simulink model "bidirectional_fixvoltage"  (R2016a)
settings: Solver=ode1  StartTime=0.0  StopTime=inf  FixedStep=1e-5  RelTol=1e-3
undefined symbols (not defined in the file): Ion, Lithium
libraries: powerlib x12, simulink x2, electricdrivelib x1
settings Model: Creator=Power Lab  LastModifiedBy=VARUN SINGH
settings DataIOCC: LimitDataPoints=on
settings DebuggingCC: AllowSymbolicDim=off
settings ModelReferenceCC: PropagateSignalLabelsOutOfModel=off
settings GRTTargetCC: GeneratePreprocessorConditionals=Use local settings

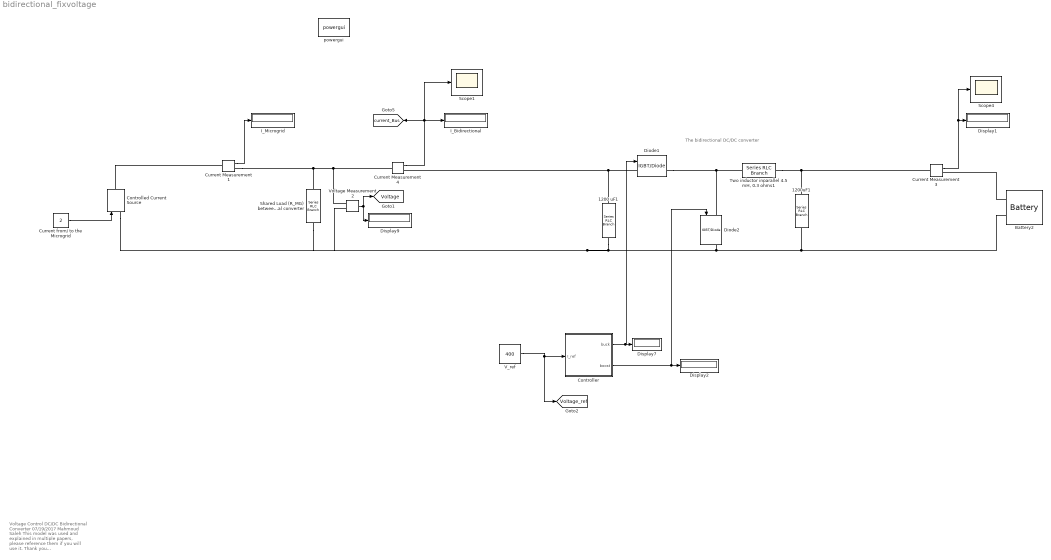
== system bidirectional_fixvoltage ==
  note: Voltage Control DC/DC Bidirectional Converter
      | 07/19/2017 Mahmoud Saleh
      | This model was used and explained in multiple papers, please reference them if you will use it. Thank you
      | ---------------------------------------------------------------------------------------------------------------------------------------------------
      |
      | http://ieeexplore.ieee.org/document/7454295/
      | OR: https://drive.google.com/open?id=0B7mblFaJhY4VcmZ5OF9ueGxPM1U
      |
      | For Citation use :
      | - M. Saleh , Y. Esa, Y. Mhandi, W. Brandauer and A. Mohamed, "Design and implementation of CCNY DC microgrid testbed,"
      | 2016 IEEE Industry Applications Society Annual Meeting, Portland, OR, 2016.
      |
      | Also This Model was used in the paper:
      | http://ieeexplore.ieee.org/abstract/document/7731870/
      | OR: https://drive.google.com/open?id=0B7mblFaJhY4VY0dXdWdqTWNmUDg
      |
      | For Citation use :
      | -M. Saleh , A. Althaibani, Y. Esa, Y. Mhandi and A. Mohamed, "Impact of clustering microgrids on their stability and resilience during blackouts,"
      | 2015 International Conference on Smart Grid and Clean Energy Technologies (ICSGCE), Offenburg, 2015, pp. 195-200.
      |
      | Also was used in the following paper:
      | https://drive.google.com/open?id=0B7mblFaJhY4VclFOR2dLcEhQYmc
      |
      | M. Saleh, Y. Esa, and A. Moahmed “Centralized Control for DC Microgrid Using Finite State Machine” accepted and to presented
      | at the 2017 IEEE Innovative Smart Grid Technologies Conference (ISGT), Washington D.C. Metro Area, USA, 23-26 April 2017.
  note: The bidirectional DC/DC converter
  1200 uF1 : powerlib/Elements/Series RLC Branch  LConnTagsString=__new0  RConnTagsString=__new0  BranchType=RC  Resistance=0.001  Inductance=3e-3  SetiL0=off  InitialCurrent=0  Capacitance=1200e-6  Setx0=off  InitialVoltage=0  Measurements=None
  1200uF1 : powerlib/Elements/Series RLC Branch  LConnTagsString=__new0  RConnTagsString=__new0  BranchType=C  Resistance=1  Inductance=3e-3  SetiL0=off  InitialCurrent=0  Capacitance=1200e-6  Setx0=off  InitialVoltage=0  Measurements=None
  Battery2 : electricdrivelib/Extra Sources/Battery  BatType=Lithium-Ion  ShowTempParam=off  ThermalPreset=no  NomV=120  NomQ=100  SOC=50  Batt_Tr=0.1  PresetModel=on  MaxQ=100  MinV=90  FullV=139.6785  Dis_rate=43.4783  R=0.012  Normal_OP=90.4348  expZone="[129.6463      4.913043]"  current=[1.5 3]  Units=Ampere-hour  Tci=20  NomT=20  T2=-30  MaxQ2=4.8  FullV2=7.1  Normal_OP2=5.72  expZone2="[6.58  1]"  Rca=0.6  ti=1000  Dp=0
  Controlled Current Source : powerlib/Electrical Sources/Controlled Current Source  Initialize=on  Source_Type=AC  Amplitude=0  Phase=0  Frequency=0  Measurements=None
  Controller : Subsystem
  Current Measurement1 : powerlib/Measurements/Current Measurement  PhasorSimulation=off  OutputType=Complex  PSBequivalent=0
  Current Measurement3 : powerlib/Measurements/Current Measurement  PhasorSimulation=off  OutputType=Complex  PSBequivalent=0
  Current Measurement4 : powerlib/Measurements/Current Measurement  PhasorSimulation=off  OutputType=Complex  PSBequivalent=0
  Current from/ to the Microgrid : Constant  Value=2
  Diode1 : powerlib/Power Electronics/IGBT//Diode  Ron=1e-3  Rs=1e5  Cs=inf  Measurements=on
  Diode2 : powerlib/Power Electronics/IGBT//Diode  Ron=1e-3  Rs=1e5  Cs=inf  Measurements=on
  Display{1..2,7,9} (4 alike) : Display
  I_Bidirectional : Display
  I_Microgrid : Display
  Scope1 : Scope
  Scope4 : Scope
  "Shared Load (R_MG) between the Microgrid and the battery through the bidirectional converter " : powerlib/Elements/Series RLC Branch  LConnTagsString=__new0  RConnTagsString=__new0  BranchType=R  Resistance=100  Inductance=3e-3  SetiL0=off  InitialCurrent=0  Capacitance=200e-6  Setx0=off  InitialVoltage=0  Measurements=None
  "Two inductor inparallel 4.5 mH, 0.3 ohms1" : powerlib/Elements/Series RLC Branch  LConnTagsString=__new0  RConnTagsString=__new0  BranchType=RL  Resistance=.25  Inductance=4.5e-3  SetiL0=off  InitialCurrent=0  Capacitance=1e-6  Setx0=off  InitialVoltage=0  Measurements=None
  V_ref : Constant  Value=400
  Voltage Measurement2 : powerlib/Measurements/Voltage Measurement  PhasorSimulation=off  OutputType=Complex  PSBequivalent=0
  powergui : powerlib/powergui  Priority=1  SimulationMode=Discrete  SolverType=Backward Euler  SampleTime=1e-5  frequency=60  SPID=off  DisableSnubberDevices=off  DisableRonSwitches=off  DisableVfSwitches=off  SwTol=0  DisplayEquations=off  Interpol=off  ExternalGateDelay=off  methode=off  Ts=0  FunctionMessages=off  echomessages=off  HookPort=off  EnableUseOfTLC=off  x0status=blocks  frequencyindice=0  Pbase=100e6  ErrMax=1e-4  Iterations=50  UnitsV=kV  UnitsW=MW  buscounter=0  RestoreLinks=warning  ResistiveCurrentMeasurement=off  Frange=[0:2:500]  Ylog=off  Xlog=on  ShowGrid=off  save=off  variable=ZData  structure=0  ZoomFFT=off  StartTime=0.0  cycles=1  DisplayStyle=1  fundamental=60  FreqAxis=off  MaxFrequency=1000  frequencyindicesteady=1  RmsSteady=1  display=off
  tag scope: Voltage=global, Voltage_ref=global, current_Bus=global
  wires:
  Current Measurement3/1 -> Display1/1, Scope4/1
  Controller/2(boost) -> Diode2/1, Display2/1
  Controller/1(buck) -> Diode1/1, Display7/1
  Current Measurement4/1 -> [current_Bus], Scope1/1, I_Bidirectional/1
  Voltage Measurement2/1 -> Display9/1, [Voltage]
  Current Measurement1/1 -> I_Microgrid/1
  V_ref/1 -> [Voltage_ref], Controller/1(I_ref)
  Current from/ to the Microgrid/1 -> Controlled Current Source/1
  connections:
  Voltage Measurement2/LConn2 -- "Shared Load (R_MG) between the Microgrid and the battery through the bidirectional converter "/RConn1 -- Controlled Current Source/LConn1 -- 1200 uF1/RConn1 -- Diode2/RConn1 -- Battery2/LConn2 -- 1200uF1/RConn1
  Diode2/LConn1 -- Diode1/RConn1 -- "Two inductor inparallel 4.5 mH, 0.3 ohms1"/LConn1
  Current Measurement3/LConn1 -- "Two inductor inparallel 4.5 mH, 0.3 ohms1"/RConn1 -- 1200uF1/LConn1
  1200 uF1/LConn1 -- Current Measurement4/RConn1 -- Diode1/LConn1
  "Shared Load (R_MG) between the Microgrid and the battery through the bidirectional converter "/LConn1 -- Current Measurement4/LConn1 -- Voltage Measurement2/LConn1 -- Current Measurement1/RConn1
  Battery2/LConn1 -- Current Measurement3/RConn1
  Controlled Current Source/RConn1 -- Current Measurement1/LConn1

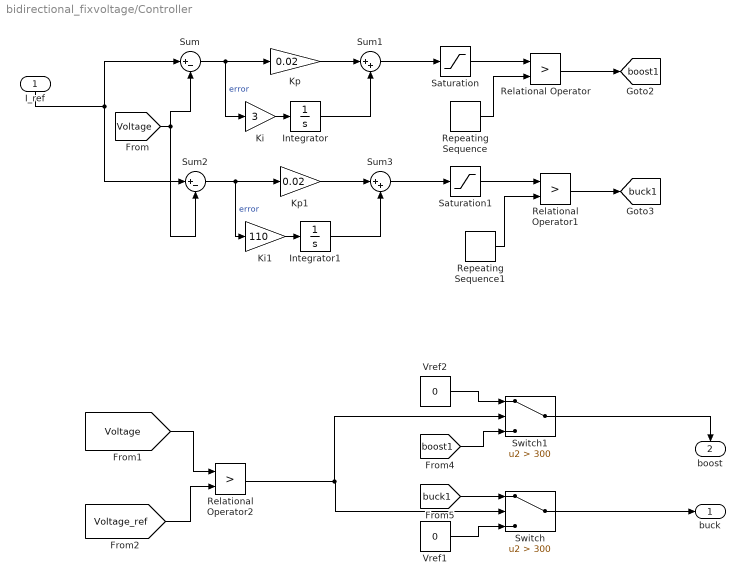
== system bidirectional_fixvoltage/Controller ==
  I_ref : Inport
  Integrator : Integrator  LimitOutput=on  UpperSaturationLimit=0.9  LowerSaturationLimit=0
  Integrator1 : Integrator  LimitOutput=on  UpperSaturationLimit=0.9  LowerSaturationLimit=0
  Ki : Gain  Gain=3
  Ki1 : Gain  Gain=110
  Kp : Gain  Gain=0.02
  Kp1 : Gain  Gain=0.02
  Relational Operator : RelationalOperator  Operator=>  OutDataTypeStr=boolean
  Relational Operator1 : RelationalOperator  Operator=>  OutDataTypeStr=boolean
  Relational Operator2 : RelationalOperator  Operator=>  OutDataTypeStr=boolean
  Repeating Sequence : simulink/Sources/Repeating Sequence  rep_seq_t=[0 1/5000]  rep_seq_y=[0 1]
  Repeating Sequence1 : simulink/Sources/Repeating Sequence  rep_seq_t=[0 1/5000]  rep_seq_y=[0 1]
  Saturation : Saturate  UpperLimit=0.9  LowerLimit=0
  Saturation1 : Saturate  UpperLimit=0.9  LowerLimit=0
  Sum : Sum  Inputs=|+-
  Sum1 : Sum  Inputs=|++
  Sum2 : Sum  Inputs=|+-
  Sum3 : Sum  Inputs=|++
  Switch : Switch  Criteria=u2 > Threshold  Threshold=300
  Switch1 : Switch  Criteria=u2 > Threshold  Threshold=300
  Vref1 : Constant  Value=0
  Vref2 : Constant  Value=0
  buck : Outport
  boost : Outport  Port=2
  tag scope: boost1=global, buck1=global
  wires:
  Switch/1 -> buck/1
  [boost1] -> Switch1/3
  Switch1/1 -> boost/1
  Ki1/1 -> Integrator1/1
  Saturation1/1 -> Relational Operator1/1
  Saturation/1 -> Relational Operator/1
  Sum2/1 -> Kp1/1, Ki1/1  "error"
  Relational Operator1/1 -> [buck1]
  Kp1/1 -> Sum3/1
  [Voltage] -> Sum2/2, Sum/2
  Repeating Sequence1/1 -> Relational Operator1/2
  Repeating Sequence/1 -> Relational Operator/2
  Integrator1/1 -> Sum3/2
  Sum3/1 -> Saturation1/1
  Ki/1 -> Integrator/1
  Sum1/1 -> Saturation/1
  I_ref/1 -> Sum/1, Sum2/1
  Relational Operator/1 -> [boost1]
  Sum/1 -> Ki/1, Kp/1  "error"
  Kp/1 -> Sum1/1
  Integrator/1 -> Sum1/2
  Vref2/1 -> Switch1/1
  Vref1/1 -> Switch/3
  [buck1] -> Switch/1
  [Voltage] -> Relational Operator2/1
  [Voltage_ref] -> Relational Operator2/2
  Relational Operator2/1 -> Switch1/2, Switch/2
